simulink model "Sl_blind_object"  (R2015a)
settings: Solver=ode45  StartTime=0.0  StopTime=2*1440  RelTol=1e-3
values from neighbouring files (symbols this model uses):
  J = 1    [Sc_blind_object.m]
  kedn = 100    [Sc_blind_object.m]
  kl = 1    [Sc_blind_object.m]
  km = 1    [Sc_blind_object.m]
  kt = 10    [Sc_blind_object.m]
  L = 1    [Sc_blind_object.m]
  R = 100    [Sc_blind_object.m]
  T = 1    [Sc_blind_object.m]
settings Model: Creator=Vladislav  LastModifiedBy=Vladislav

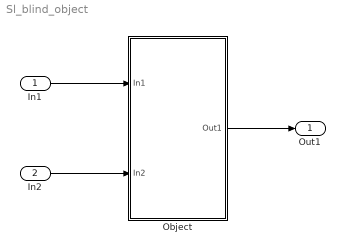
== system Sl_blind_object ==
  In1 : Inport
  In2 : Inport  Port=2
  Object : Subsystem
  Out1 : Outport
  wires:
  In2/1 -> Object/2(In2)
  In1/1 -> Object/1(In1)
  Object/1(Out1) -> Out1/1

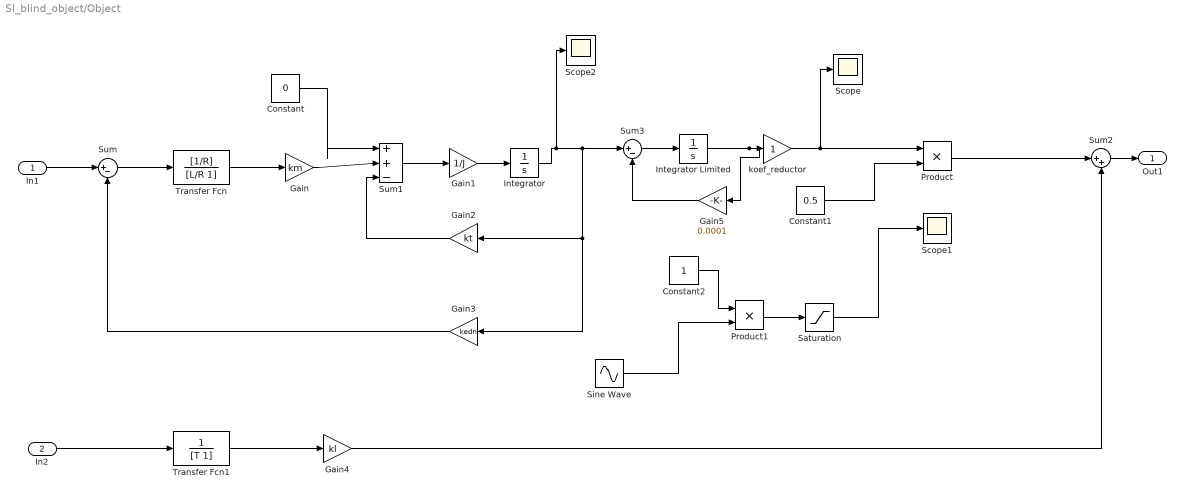
== system Sl_blind_object/Object ==
  In1 : Inport
  In2 : Inport  Port=2
  Constant : Constant  Value=0
  Constant1 : Constant  Value=0.5
  Constant2 : Constant
  Gain : Gain  Gain=km
  Gain1 : Gain  Gain=1/J
  Gain2 : Gain  Gain=kt
  Gain3 : Gain  Gain=kedn
  Gain4 : Gain  Gain=kl
  Gain5 : Gain  Gain=0.0001
  Integrator : Integrator
  Integrator Limited : Integrator  LimitOutput=on  UpperSaturationLimit=1  LowerSaturationLimit=0  IgnoreLimit=on
  Product : Product
  Product1 : Product
  Saturation : Saturate  UpperLimit=Inf  LowerLimit=0
  Scope : Scope
  Scope1 : Scope
      settings: SaveName=ScopeData2
  Scope2 : Scope
      settings: SaveName=ScopeData3
  Sine Wave : Sin  Amplitude=0.5  Bias=0.5  Frequency=1/1440*2*pi  SampleTime=0
  Sum : Sum  Inputs=|+-
  Sum1 : Sum  Inputs=|++-
  Sum2 : Sum  Inputs=|++
  Sum3 : Sum  Inputs=|+-
  Transfer Fcn : TransferFcn  Numerator=[1/R]  Denominator=[L/R 1]
  Transfer Fcn1 : TransferFcn  Denominator=[T 1]
  koef_reductor : Gain
  Out1 : Outport
  wires:
  Transfer Fcn/1 -> Gain/1
  In2/1 -> Transfer Fcn1/1
  Product1/1 -> Saturation/1
  Sum/1 -> Transfer Fcn/1
  Sum1/1 -> Gain1/1
  Gain1/1 -> Integrator/1
  koef_reductor/1 -> Product/1, Scope/1
  In1/1 -> Sum/1
  Gain/1 -> Sum1/2
  Constant/1 -> Sum1/1
  Integrator Limited/1 -> Gain5/1, koef_reductor/1
  Gain3/1 -> Sum/2
  Gain2/1 -> Sum1/3
  Product/1 -> Sum2/1
  Integrator/1 -> Scope2/1, Sum3/1, Gain3/1, Gain2/1
  Sine Wave/1 -> Product1/2
  Saturation/1 -> Scope1/1
  Transfer Fcn1/1 -> Gain4/1
  Sum2/1 -> Out1/1
  Constant1/1 -> Product/2
  Gain4/1 -> Sum2/2
  Constant2/1 -> Product1/1
  Sum3/1 -> Integrator Limited/1
  Gain5/1 -> Sum3/2
